simulink model "hruchevo"  (R2021b)
settings: Solver=VariableStepAuto  StartTime=0.0  StopTime=10.0  RelTol=1e-3
settings Model: Creator=Семенов Никита  LastModifiedBy=Семенов Никита

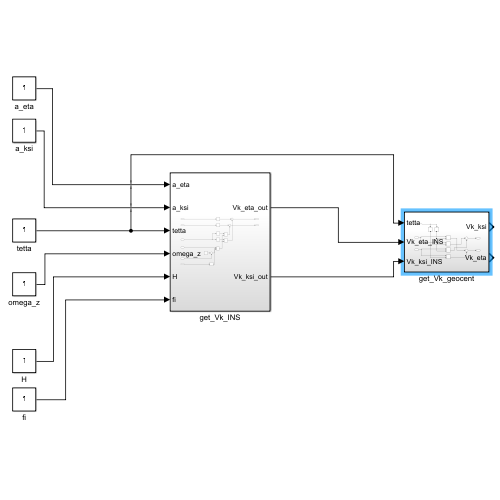
[thumbnail: Simulink's stored preview of the top-level diagram]
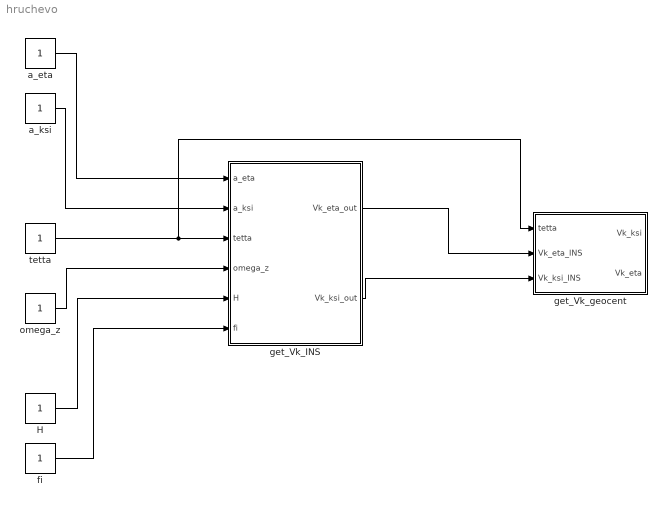
== system hruchevo ==
  H : Constant
  a_eta : Constant
  a_ksi : Constant
  fi : Constant
  get_Vk_INS : Subsystem
  get_Vk_geocent : Subsystem
  omega_z : Constant
  tetta : Constant
  wires:
  a_eta/1 -> get_Vk_INS/1(a_eta)
  a_ksi/1 -> get_Vk_INS/2(a_ksi)
  tetta/1 -> get_Vk_geocent/1(tetta), get_Vk_INS/3(tetta)
  omega_z/1 -> get_Vk_INS/4(omega_z)
  H/1 -> get_Vk_INS/5(H)
  fi/1 -> get_Vk_INS/6(fi)
  get_Vk_INS/1(Vk_eta_out) -> get_Vk_geocent/2(Vk_eta_INS)
  get_Vk_INS/2(Vk_ksi_out) -> get_Vk_geocent/3(Vk_ksi_INS)

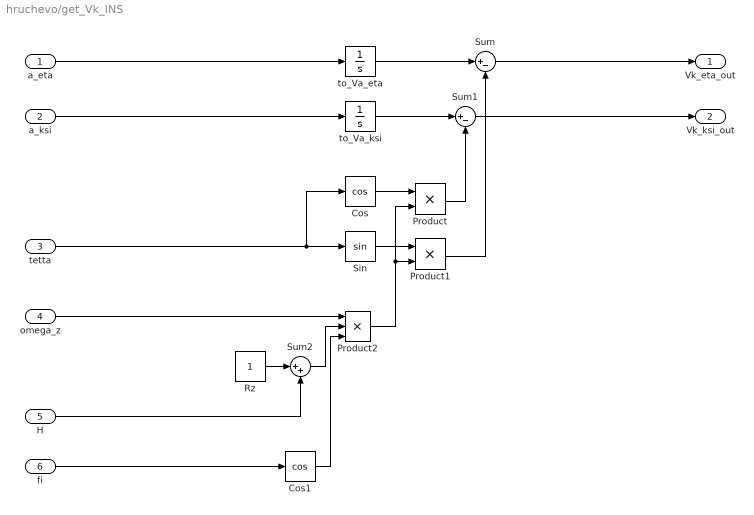
== system hruchevo/get_Vk_INS ==
  a_eta : Inport
  a_ksi : Inport  Port=2
  tetta : Inport  Port=3
  omega_z : Inport  Port=4
  H : Inport  Port=5
  fi : Inport  Port=6
  Cos : Trigonometry  Operator=cos
  Cos1 : Trigonometry  Operator=cos
  Product : Product
  Product1 : Product
  Product2 : Product  Inputs=3
  Rz : Constant
  Sin : Trigonometry
  Sum : Sum  Inputs=|+-
  Sum1 : Sum  Inputs=|+-
  Sum2 : Sum  Inputs=|++
  to_Va_eta : Integrator
  to_Va_ksi : Integrator
  Vk_eta_out : Outport
  Vk_ksi_out : Outport  Port=2
  wires:
  Sin/1 -> Product1/1
  to_Va_ksi/1 -> Sum1/1
  Rz/1 -> Sum2/1
  tetta/1 -> Sin/1, Cos/1
  H/1 -> Sum2/2
  a_ksi/1 -> to_Va_ksi/1
  Sum2/1 -> Product2/2
  fi/1 -> Cos1/1
  Sum1/1 -> Vk_ksi_out/1
  Product1/1 -> Sum/2
  Product/1 -> Sum1/2
  to_Va_eta/1 -> Sum/1
  a_eta/1 -> to_Va_eta/1
  Cos1/1 -> Product2/3
  Cos/1 -> Product/1
  omega_z/1 -> Product2/1
  Product2/1 -> Product/2, Product1/2
  Sum/1 -> Vk_eta_out/1

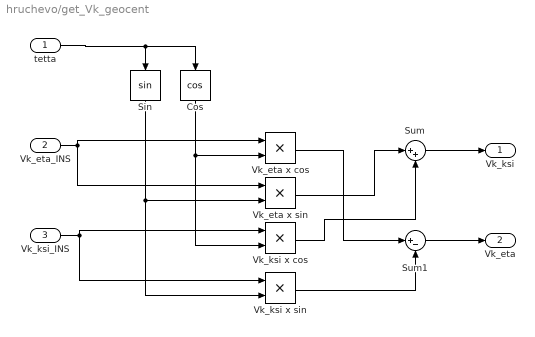
== system hruchevo/get_Vk_geocent ==
  tetta : Inport
  Vk_eta_INS : Inport  Port=2
  Vk_ksi_INS : Inport  Port=3
  Cos : Trigonometry  Operator=cos
  Sin : Trigonometry
  Sum : Sum  Inputs=|++
  Sum1 : Sum  Inputs=|+-
  Vk_eta x cos : Product
  Vk_eta x sin : Product
  Vk_ksi x cos : Product
  Vk_ksi x sin : Product
  Vk_ksi : Outport
  Vk_eta : Outport  Port=2
  wires:
  Vk_ksi_INS/1 -> Vk_ksi x sin/1, Vk_ksi x cos/1
  tetta/1 -> Cos/1, Sin/1
  Sum1/1 -> Vk_eta/1
  Cos/1 -> Vk_ksi x cos/2, Vk_eta x cos/2
  Vk_eta_INS/1 -> Vk_eta x cos/1, Vk_eta x sin/1
  Vk_ksi x sin/1 -> Sum1/2
  Sin/1 -> Vk_ksi x sin/2, Vk_eta x sin/2
  Vk_eta x sin/1 -> Sum/1
  Vk_ksi x cos/1 -> Sum/2
  Vk_eta x cos/1 -> Sum1/1
  Sum/1 -> Vk_ksi/1
